simulink model "goloole"  (Simulink 7.8)
settings: Solver=ode45  StartTime=0.0  StopTime=10.0  RelTol=1e-3
libraries: simulink x1
settings Model: Creator=nike  LastModifiedBy=nike

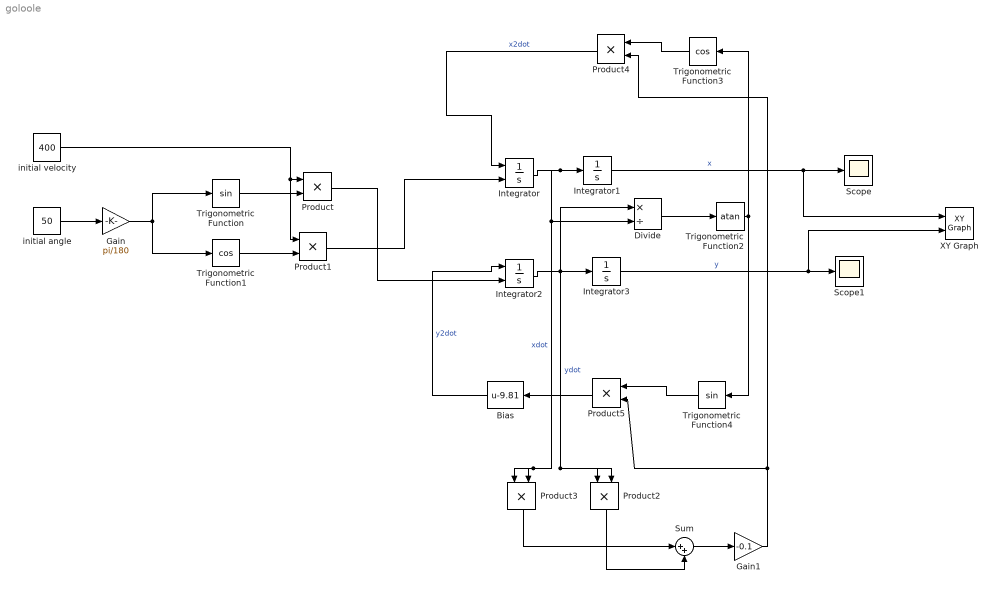
== system goloole ==
  Bias : Bias  Bias=-9.81
  Divide : Product  Inputs=*/
  Gain : Gain  Gain=pi/180
  Gain1 : Gain  Gain=-0.1
  Integrator : Integrator  InitialConditionSource=external
  Integrator1 : Integrator
  Integrator2 : Integrator  InitialConditionSource=external
  Integrator3 : Integrator
  Product{,1..5} (6 alike) : Product  RndMeth=Zero
  Scope : Scope
  Scope1 : Scope
  Sum : Sum  Inputs=|++
  Trigonometric Function : Trigonometry
  Trigonometric Function1 : Trigonometry  Operator=cos
  Trigonometric Function2 : Trigonometry  Operator=atan
  Trigonometric Function3 : Trigonometry  Operator=cos
  Trigonometric Function4 : Trigonometry
  XY Graph : simulink/Sinks/XY Graph  xmin=-1  xmax=45  ymin=-1  ymax=30  st=-1
  initial angle : Constant  Value=50
  initial velocity : Constant  Value=400
  wires:
  Product4/1 -> Integrator/1  "x2dot"
  Integrator/1 -> Integrator1/1, Divide/2, Product3/1, Product3/2  "xdot"
  Integrator1/1 -> Scope/1, XY Graph/1  "x"
  Integrator2/1 -> Integrator3/1, Divide/1, Product2/2, Product2/1  "ydot"
  Integrator3/1 -> Scope1/1, XY Graph/2  "y"
  Bias/1 -> Integrator2/1  "y2dot"
  initial velocity/1 -> Product/1, Product1/1
  initial angle/1 -> Gain/1
  Gain/1 -> Trigonometric Function/1, Trigonometric Function1/1
  Trigonometric Function/1 -> Product/2
  Trigonometric Function1/1 -> Product1/2
  Product1/1 -> Integrator/2
  Product/1 -> Integrator2/2
  Divide/1 -> Trigonometric Function2/1
  Trigonometric Function2/1 -> Trigonometric Function3/1, Trigonometric Function4/1
  Product3/1 -> Sum/1
  Product2/1 -> Sum/2
  Sum/1 -> Gain1/1
  Trigonometric Function3/1 -> Product4/1
  Gain1/1 -> Product4/2, Product5/2
  Trigonometric Function4/1 -> Product5/1
  Product5/1 -> Bias/1
